simulink model "simulink_q4_JM_v2"  (R2024b)
settings: Solver=ode4  StartTime=0.0  StopTime=TF  RelTol=1e-3
values from neighbouring files (symbols this model uses):
  U0 = [0.525841853692 -0.00469375602825 0 0 0]    [ICs_aircraft2_180Kts_CG1.mat]    (also in ICs_aircraft2_180Kts_CG2.mat = [0.525939752377 -0.00596702425354 0 0 0]; ICs_aircraft2_75Kts_CG1.mat = [0.0938327586982 -0.025121721174 0 0 0]; ICs_aircraft2_75Kts_CG2.mat = [0.0933937108451 -0.0325384431522 0 0 0])
undefined symbols (not defined in the file or in its folder): q3d, q3i, q3n, q3p, V_trim
libraries: cstblocks x7, slpidlib x1
settings Model: Creator=Bez  LastModifiedBy=Bez

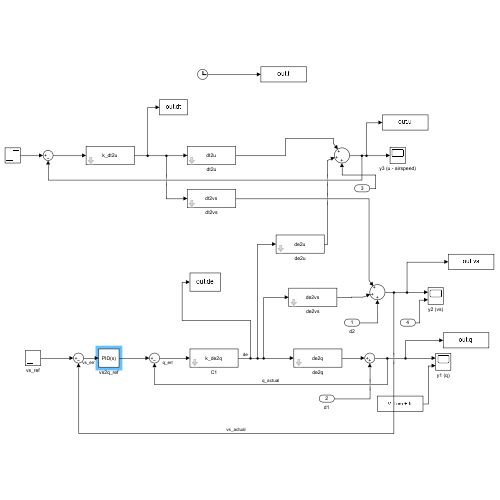
[thumbnail: Simulink's stored preview of the top-level diagram]
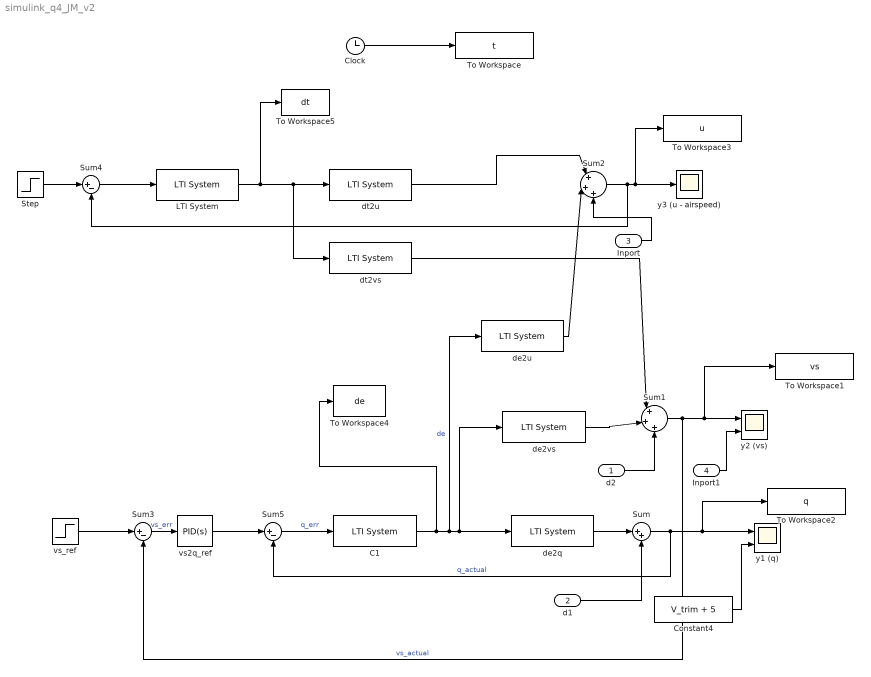
== system simulink_q4_JM_v2 ==
  d2 : Inport
  d1 : Inport  Port=2
  Inport : Inport  Port=3
  Inport1 : Inport  Port=4
  C1 : cstblocks/LTI System  sys=k_de2q  IC=[]  PadeOrder=0
  Clock : Clock
  Constant4 : Constant  Value=V_trim + 5
  LTI System : cstblocks/LTI System  sys=k_dt2u  IC=[]  PadeOrder=0
  Step : Step  Before=U0(1,:)  After=8.3  SampleTime=0.01
  Sum : Sum  Inputs=|++
  Sum1 : Sum  Inputs=|+|+|+
  Sum2 : Sum  Inputs=|+|+|+
  Sum3 : Sum  Inputs=|+-
  Sum4 : Sum  Inputs=|+-
  Sum5 : Sum  Inputs=|+-
  To Workspace : ToWorkspace  VariableName=t  SampleTime=-1
  To Workspace1 : ToWorkspace  VariableName=vs  SampleTime=-1
  To Workspace2 : ToWorkspace  VariableName=q  SampleTime=-1
  To Workspace3 : ToWorkspace  VariableName=u  SampleTime=-1
  To Workspace4 : ToWorkspace  VariableName=de  SampleTime=-1
  To Workspace5 : ToWorkspace  VariableName=dt  SampleTime=-1
  de2q : cstblocks/LTI System  sys=de2q  IC=[]  PadeOrder=0
  de2u : cstblocks/LTI System  sys=de2u  IC=[]  PadeOrder=0
  de2vs : cstblocks/LTI System  sys=de2vs  IC=[]  PadeOrder=0
  dt2u : cstblocks/LTI System  sys=dt2u  IC=[]  PadeOrder=0
  dt2vs : cstblocks/LTI System  sys=dt2vs  IC=[]  PadeOrder=0
  vs2q_ref : slpidlib/PID Controller  Controller=PID  Form=Parallel  TimeDomain=Continuous-time  UseExternalTs=off  SampleTime=-1  IntegratorMethod=Forward Euler  FilterMethod=Forward Euler  ControllerParametersSource=internal  P=q3p  I=q3i  UseKiTs=off  D=q3d  UseExternalDerivativeSource=off  N=q3n  UseFilter=on  TunerSelectOption=Transfer Function Based (PID Tuner App)  InitialConditionSource=internal  InitialConditionForIntegrator=0  InitialConditionForFilter=0  DifferentiatorICPrevScaledInput=0  ExternalReset=none  TrackingMode=off  Kt=1  LimitOutput=off  SatLimitsSource=internal  UpperSaturationLimit=inf  LowerSaturationLimit=-inf  LinearizeAsGain=on  AntiWindupMode=none  Kb=1  LimitIntegrator=off  UpperIntegratorSaturationLimit=inf  LowerIntegratorSaturationLimit=-inf  POutMin=[]  POutMax=[]  IOutMin=[]  IOutMax=[]  DOutMin=[]  DOutMax=[]  NOutMin=[]  NOutMax=[]  SumOutMin=[]  SumOutMax=[]  SaturationOutMin=[]  SaturationOutMax=[]  PParamMin=[]  PParamMax=[]  IParamMin=[]  IParamMax=[]  DParamMin=[]  DParamMax=[]  NParamMin=[]  NParamMax=[]  KbParamMin=[]  KbParamMax=[]  KtParamMin=[]  KtParamMax=[]  KbOutMin=[]  KbOutMax=[]  KtOutMin=[]  KtOutMax=[]  IntegratorOutMin=[]  IntegratorOutMax=[]  FilterOutMin=[]  FilterOutMax=[]  SumI1OutMin=[]  SumI1OutMax=[]  SumI2OutMin=[]  SumI2OutMax=[]  SumI3OutMin=[]  SumI3OutMax=[]  SumI4OutMin=[]  SumI4OutMax=[]  SumDOutMin=[]  SumDOutMax=[]  DifferentiatorOutMin=[]  DifferentiatorOutMax=[]  FilterDiffOutCoefMin=[]  FilterDiffOutCoefMax=[]  ReciprocalOutMin=[]  ReciprocalOutMax=[]  SumDenOutMin=[]  SumDenOutMax=[]  SumNumOutMin=[]  SumNumOutMax=[]  DivideOutMin=[]  DivideOutMax=[]  UdiffTsProdOutMin=[]  UdiffTsProdOutMax=[]  NTsProdOutMin=[]  NTsProdOutMax=[]  UintegralTsProdOutMin=[]  UintegralTsProdOutMax=[]  UngainTsProdOutMin=[]  UngainTsProdOutMax=[]  ClampingZeroOutDataTypeStr=Inherit: Inherit via back propagation  ClampingZeroOutMin=[]  ClampingZeroOutMax=[]  FilterDenConstantOutDataTypeStr=Inherit: Inherit via back propagation  FilterDenConstantOutMin=[]  FilterDenConstantOutMax=[]  PCopyOutDataTypeStr=Inherit: Inherit via back propagation  PCopyOutMin=[]  PCopyOutMax=[]  NCopyOutDataTypeStr=Inherit: Inherit via back propagation  NCopyOutMin=[]  NCopyOutMax=[]  IntegratorContinuousStateAttributes=''  IntegratorStateMustResolveToSignalObject=off  IntegratorRTWStateStorageClass=Auto  FilterContinuousStateAttributes=''  FilterStateMustResolveToSignalObject=off  FilterRTWStateStorageClass=Auto  ParallelPVariant=InternalParameters  IdealPVariant=Disabled  IVariant=InternalParameters  DVariant=InternalParameters  IntegratorVariant=Continuous  SatVariant=Disabled  AWVariant=Passthrough  PCopyVariant=Disabled  TRVariant=Disabled  FdbkBlocksVariant=Forward  IdealPFdbkVariant=Disabled  SatFdbkVariant=Disabled  DerivativeFilterVariant=ContFilter  NVariant=InternalParameters  NCopyVariant=Disabled  FilterICVariant=InternalICsFilter  IntegratorICVariant=InternalICs  ExternalResetVariant=Disabled  TRSumVariant=Passthrough  SumFdbkVariant=Disabled  SumVariant=Sum_PID  TsampFilterVariant=InternalTs  TsampNgainVariant=Passthrough  TsampIntegralVariant=Passthrough  ExternalSaturationOutDataTypeStr=Inherit: Same as second input  DerivativeSourceVariant=ErrorSignal  PreIntVariant=InternalPreInt
  vs_ref : Step  Before=U0(2,:)  After=8.3  SampleTime=0.01
  y1 (q) : Scope  NumInputPorts=2
  y2 (vs) : Scope  NumInputPorts=2
  y3 (u - airspeed) : Scope
  wires:
  Sum3/1 -> vs2q_ref/1  "vs_err"
  vs2q_ref/1 -> Sum5/1
  C1/1 -> de2vs/1, de2q/1, de2u/1, To Workspace4/1  "de"
  de2vs/1 -> Sum1/2
  Sum1/1 -> To Workspace1/1, y2 (vs)/1, Sum3/2  "vs_actual"
  Inport/1 -> Sum2/3
  dt2u/1 -> Sum2/1
  d2/1 -> Sum1/3
  Sum/1 -> To Workspace2/1, y1 (q)/1, Sum5/2  "q_actual"
  de2q/1 -> Sum/1
  Sum2/1 -> To Workspace3/1, y3 (u - airspeed)/1, Sum4/2
  Clock/1 -> To Workspace/1
  Inport1/1 -> y2 (vs)/2
  Constant4/1 -> y1 (q)/2
  vs_ref/1 -> Sum3/1
  Sum5/1 -> C1/1  "q_err"
  d1/1 -> Sum/2
  de2u/1 -> Sum2/2
  dt2vs/1 -> Sum1/1
  LTI System/1 -> To Workspace5/1, dt2vs/1, dt2u/1
  Step/1 -> Sum4/1
  Sum4/1 -> LTI System/1
